simulink model "C172S_RollAttitudeHold_V1"  (R2026a)
settings: Solver=ode4  StartTime=0  StopTime=40  FixedStep=0.01
InitFcn:
  | rah1Data = c172sLateralDirectionalData();
  | [~,rah1Plant] = c172sLateralDirectionalPlant(rah1Data);
  | rah1YawController = c172sYawDamperData();
  | rah1RudderActuator = c172sRudderActuatorData();
  | rah1Controller = c172sRollAttitudeControllerData();
  | rah1AileronActuator = c172sAileronActuatorData();
  | if ~strcmp(rah1Data.model.version,rah1Controller.requiredPlantVersion), error('RAH V1 plant dependency mismatch.'); end
  | if ~strcmp(rah1YawController.artifactRevision,rah1Controller.requiredYawDamperRevision), error('RAH V1 yaw-controller dependency mismatch.'); end
  | if ~strcmp(rah1RudderActuator.artifactRevision,rah1Controller.requiredRudderAuditRevision), error('RAH V1 rudder-audit dependency mismatch.'); end
  | if ~strcmp(rah1AileronActuator.artifactRevision,rah1Controller.requiredAileronAuditRevision), error('RAH V1 aileron-audit dependency mismatch.'); end
  | A_rah1 = rah1Plant.A; B_rah1 = rah1Plant.B;
  | C_rah1 = rah1Plant.C; D_rah1 = rah1Plant.D;
  | Kphi_rah1 = rah1Controller.bankProportionalGain;
  | Ki_rah1 = rah1Controller.bankIntegralGain_per_s;
  | Kp_rah1 = rah1Controller.rollRateGain_s;
  | Tcmd_rah1 = rah1Controller.commandFilterTimeConstant_s;
  | Kr_rah1 = rah1YawController.rudderGain_s;
  | Tw_rah1 = rah1YawController.washoutTimeConstant_s;
  | TsRudder_rah1 = rah1RudderActuator.sensor.filterTimeConstant_s;
  | tauRudder_rah1 = rah1RudderActuator.dynamics.timeConstant_s;
  | TsRoll_rah1 = rah1AileronActuator.sensor.filterTimeConstant_s;
  | tauAileron_rah1 = rah1AileronActuator.dynamics.timeConstant_s;
  | Tt_rah1 = rah1AileronActuator.antiWindup.trackingTimeConstant_s;
  | delaySampleTime_rah1 = rah1AileronActuator.sensor.nominalDelay_s;
  | bankCommandLower_rah1_rad = rah1Controller.commandAuthority.lowerLimit_rad;
  | bankCommandUpper_rah1_rad = rah1Controller.commandAuthority.upperLimit_rad;
  | autoAileronLower_rah1_rad = rah1AileronActuator.authority.lowerLimit_rad;
  | autoAileronUpper_rah1_rad = rah1AileronActuator.authority.upperLimit_rad;
  | aileronRateLower_rah1_radps = -deg2rad(rah1AileronActuator.dynamics.rateLimit_degps);
  | aileronRateUpper_rah1_radps = deg2rad(rah1AileronActuator.dynamics.rateLimit_degps);
  | totalAileronLower_rah1_rad = rah1AileronActuator.physicalTravel.lowerLimit_rad;
  | totalAileronUpper_rah1_rad = rah1AileronActuator.physicalTravel.upperLimit_rad;
  | autoRudderLower_rah1_rad = rah1RudderActuator.authority.lowerLimit_rad;
  | autoRudderUpper_rah1_rad = rah1RudderActuator.authority.upperLimit_rad;
  | rudderRateLower_rah1_radps = -deg2rad(rah1RudderActuator.dynamics.rateLimit_degps);
  | rudderRateUpper_rah1_radps = deg2rad(rah1RudderActuator.dynamics.rateLimit_degps);
  | totalRudderLower_rah1_rad = rah1RudderActuator.physicalTravel.lowerLimit_rad;
  | totalRudderUpper_rah1_rad = rah1RudderActuator.physicalTravel.upperLimit_rad;
  | if ~exist('bankCommand_rah1_rad','var'), bankCommand_rah1_rad = deg2rad(10); end
  | if ~exist('pilotAileronBias_rah1_rad','var'), pilotAileronBias_rah1_rad = 0; end
  | if ~exist('pilotAileronPulse_rah1_rad','var'), pilotAileronPulse_rah1_rad = 0; end
  | if ~exist('pilotRudderBias_rah1_rad','var'), pilotRudderBias_rah1_rad = 0; end
  | if ~exist('pilotRudderPulse_rah1_rad','var'), pilotRudderPulse_rah1_rad = 0; end
  | if ~exist('aileronPulseStart_rah1_s','var'), aileronPulseStart_rah1_s = 5; end
  | if ~exist('aileronPulseEnd_rah1_s','var'), aileronPulseEnd_rah1_s = 6; end
  | if ~exist('rudderPulseStart_rah1_s','var'), rudderPulseStart_rah1_s = 5; end
  | if ~exist('rudderPulseEnd_rah1_s','var'), rudderPulseEnd_rah1_s = 6; end
  | if ~exist('pNoiseAmplitude_rah1_radps','var'), pNoiseAmplitude_rah1_radps = 0; end
  | if ~exist('pNoiseFrequency_rah1_radps','var'), pNoiseFrequency_rah1_radps = 50; end
  | if ~exist('phiNoiseAmplitude_rah1_rad','var'), phiNoiseAmplitude_rah1_rad = 0; end
  | if ~exist('phiNoiseFrequency_rah1_radps','var'), phiNoiseFrequency_rah1_radps = 5; end
  | if ~exist('yawNoiseAmplitude_rah1_radps','var'), yawNoiseAmplitude_rah1_radps = 0; end
  | if ~exist('yawNoiseFrequency_rah1_radps','var'), yawNoiseFrequency_rah1_radps = 50; end
  | if ~exist('antiWindupEnable_rah1','var'), antiWindupEnable_rah1 = 1; end
  | if ~exist('x0_rah1','var'), x0_rah1 = zeros(5,1); end
  | if ~exist('rDelay0_rah1_radps','var'), rDelay0_rah1_radps = x0_rah1(3); end
  | if ~exist('pDelay0_rah1_radps','var'), pDelay0_rah1_radps = x0_rah1(2); end
  | if ~exist('phiDelay0_rah1_rad','var'), phiDelay0_rah1_rad = x0_rah1(4); end
  | if ~exist('rSensor0_rah1_radps','var'), rSensor0_rah1_radps = 0; end
  | if ~exist('xw0_rah1_radps','var'), xw0_rah1_radps = 0; end
  | if ~exist('deltaRAuto0_rah1_rad','var'), deltaRAuto0_rah1_rad = 0; end
  | if ~exist('pSensor0_rah1_radps','var'), pSensor0_rah1_radps = 0; end
  | if ~exist('phiSensor0_rah1_rad','var'), phiSensor0_rah1_rad = 0; end
  | if ~exist('xi0_rah1_rad_s','var'), xi0_rah1_rad_s = 0; end
  | if ~exist('deltaAAuto0_rah1_rad','var'), deltaAAuto0_rah1_rad = 0; end
  | if ~exist('filteredCommand0_rah1_rad','var'), filteredCommand0_rah1_rad = 0; end
undefined symbols (not defined in the file or in its folder): aileronPulseEnd_rah1_s, aileronPulseStart_rah1_s, antiWindupEnable_rah1, deltaAAuto0_rah1_rad, deltaRAuto0_rah1_rad, filteredCommand0_rah1_rad, pDelay0_rah1_radps, phiDelay0_rah1_rad, phiNoiseAmplitude_rah1_rad, phiNoiseFrequency_rah1_radps, phiSensor0_rah1_rad, pilotAileronBias_rah1_rad, pilotAileronPulse_rah1_rad, pilotRudderBias_rah1_rad, pilotRudderPulse_rah1_rad, pNoiseAmplitude_rah1_radps, pNoiseFrequency_rah1_radps, pSensor0_rah1_radps, rDelay0_rah1_radps, rSensor0_rah1_radps, rudderPulseEnd_rah1_s, rudderPulseStart_rah1_s, x0_rah1, xi0_rah1_rad_s, xw0_rah1_radps, yawNoiseAmplitude_rah1_radps, yawNoiseFrequency_rah1_radps
settings Model: Creator=Shahi  LastModifiedBy=Shahi

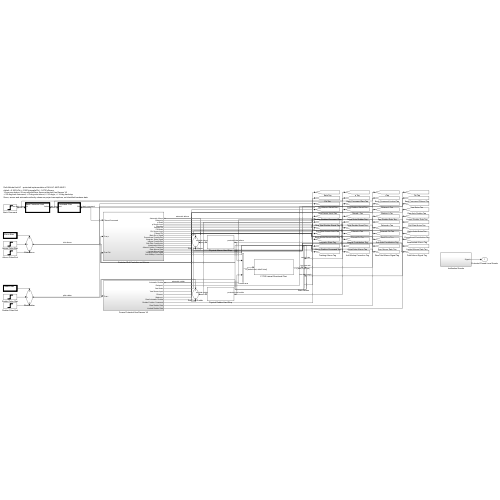
[thumbnail: Simulink's stored preview of the top-level diagram]
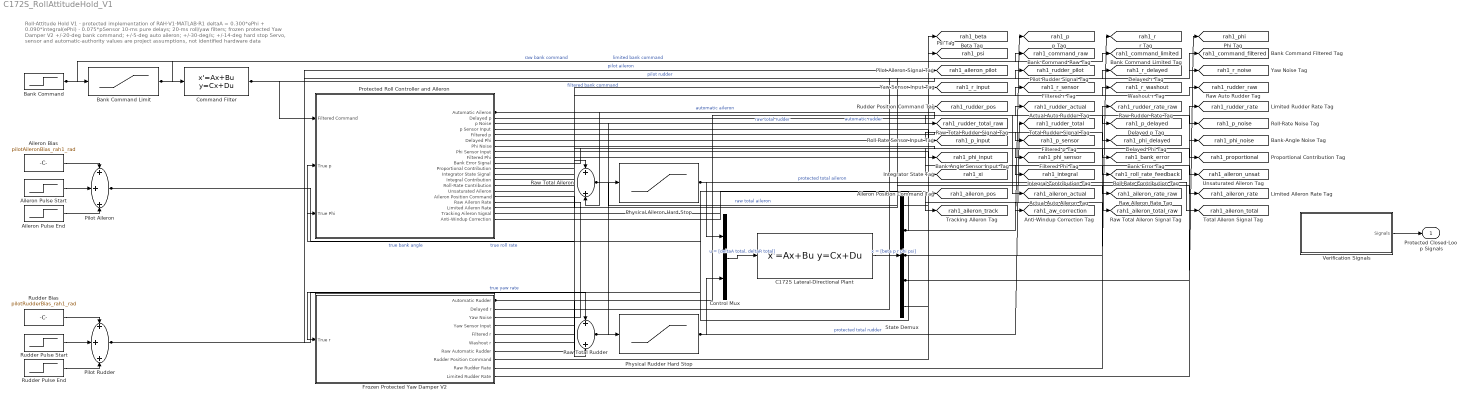
== system C172S_RollAttitudeHold_V1 ==
  note: Roll-Attitude Hold V1 - protected implementation of RAH-V1-MATLAB-R1
      | deltaA = 0.300*ePhi + 0.090*integral(ePhi) - 0.075*pSensor
      | 10-ms pure delays; 20-ms roll/yaw filters; frozen protected Yaw Damper V2
      | +/-20-deg bank command; +/-5-deg auto aileron; +/-30-deg/s; +/-14-deg hard stop
      | Servo, sensor and automatic-authority values are project assumptions, not identified hardware data
  Aileron Bias : Constant  Value=pilotAileronBias_rah1_rad
  Aileron Pulse End : Step  Time=aileronPulseEnd_rah1_s  FinalValue=-pilotAileronPulse_rah1_rad  SampleTime=0
  Aileron Pulse Start : Step  Time=aileronPulseStart_rah1_s  FinalValue=pilotAileronPulse_rah1_rad  SampleTime=0
  Bank Command : Step  Time=0  FinalValue=bankCommand_rah1_rad  SampleTime=0
  Bank Command Limit : Saturate  UpperLimit=bankCommandUpper_rah1_rad  LowerLimit=bankCommandLower_rah1_rad
  C172S Lateral-Directional Plant : StateSpace  A=A_rah1  B=B_rah1  C=C_rah1  D=D_rah1  InitialCondition=x0_rah1
  Command Filter : StateSpace  A=-1/Tcmd_rah1  B=1/Tcmd_rah1  D=0  InitialCondition=filteredCommand0_rah1_rad
  Control Mux : Mux  Inputs=2
  Frozen Protected Yaw Damper V2 : Subsystem
  Physical Aileron Hard Stop : Saturate  UpperLimit=totalAileronUpper_rah1_rad  LowerLimit=totalAileronLower_rah1_rad
  Physical Rudder Hard Stop : Saturate  UpperLimit=totalRudderUpper_rah1_rad  LowerLimit=totalRudderLower_rah1_rad
  Pilot Aileron : Sum  Inputs=+++
  Pilot Rudder : Sum  Inputs=+++
  Protected Roll Controller and Aileron : Subsystem
  Raw Total Aileron : Sum
  Raw Total Rudder : Sum
  Rudder Bias : Constant  Value=pilotRudderBias_rah1_rad
  Rudder Pulse End : Step  Time=rudderPulseEnd_rah1_s  FinalValue=-pilotRudderPulse_rah1_rad  SampleTime=0
  Rudder Pulse Start : Step  Time=rudderPulseStart_rah1_s  FinalValue=pilotRudderPulse_rah1_rad  SampleTime=0
  State Demux : Demux  Outputs=5
  Verification Signals : Subsystem
  Protected Closed-Loop Signals : Outport
  tag scope: rah1_aileron_actual=global, rah1_aileron_pilot=global, rah1_aileron_pos=global, rah1_aileron_rate=global, rah1_aileron_rate_raw=global, rah1_aileron_total=global, rah1_aileron_total_raw=global, rah1_aileron_track=global, rah1_aileron_unsat=global, rah1_aw_correction=global, rah1_bank_error=global, rah1_beta=global, rah1_command_filtered=global, rah1_command_limited=global, rah1_command_raw=global, rah1_integral=global, rah1_p=global, rah1_p_delayed=global, rah1_p_input=global, rah1_p_noise=global, rah1_p_sensor=global, rah1_phi=global, rah1_phi_delayed=global, rah1_phi_input=global, rah1_phi_noise=global, rah1_phi_sensor=global, rah1_proportional=global, rah1_psi=global, rah1_r=global, rah1_r_delayed=global, rah1_r_input=global, rah1_r_noise=global, rah1_r_sensor=global, rah1_r_washout=global, rah1_roll_rate_feedback=global, rah1_rudder_actual=global, rah1_rudder_pilot=global, rah1_rudder_pos=global, rah1_rudder_rate=global, rah1_rudder_rate_raw=global, rah1_rudder_raw=global, rah1_rudder_total=global, rah1_rudder_total_raw=global, rah1_xi=global
  wires:
  Bank Command/1 -> Bank Command Limit/1, [rah1_command_raw]  "raw bank command"
  Bank Command Limit/1 -> Command Filter/1, [rah1_command_limited]  "limited bank command"
  Command Filter/1 -> Protected Roll Controller and Aileron/1(Filtered Command), [rah1_command_filtered]  "filtered bank command"
  Aileron Bias/1 -> Pilot Aileron/1
  Aileron Pulse Start/1 -> Pilot Aileron/2
  Aileron Pulse End/1 -> Pilot Aileron/3
  Rudder Bias/1 -> Pilot Rudder/1
  Rudder Pulse Start/1 -> Pilot Rudder/2
  Rudder Pulse End/1 -> Pilot Rudder/3
  Pilot Aileron/1 -> Raw Total Aileron/1, [rah1_aileron_pilot]  "pilot aileron"
  Protected Roll Controller and Aileron/1(Automatic Aileron) -> Raw Total Aileron/2, [rah1_aileron_actual]  "automatic aileron"
  Raw Total Aileron/1 -> Physical Aileron Hard Stop/1, [rah1_aileron_total_raw]  "raw total aileron"
  Physical Aileron Hard Stop/1 -> Control Mux/1, [rah1_aileron_total]  "protected total aileron"
  Pilot Rudder/1 -> Raw Total Rudder/1, [rah1_rudder_pilot]  "pilot rudder"
  Frozen Protected Yaw Damper V2/1(Automatic Rudder) -> Raw Total Rudder/2, [rah1_rudder_actual]  "automatic rudder"
  Raw Total Rudder/1 -> Physical Rudder Hard Stop/1, [rah1_rudder_total_raw]  "raw total rudder"
  Physical Rudder Hard Stop/1 -> Control Mux/2, [rah1_rudder_total]  "protected total rudder"
  Control Mux/1 -> C172S Lateral-Directional Plant/1  "u = [deltaA total, deltaR total]"
  C172S Lateral-Directional Plant/1 -> State Demux/1  "x = [beta p r phi psi]"
  State Demux/2 -> Protected Roll Controller and Aileron/2(True p), [rah1_p]  "true roll rate"
  State Demux/4 -> Protected Roll Controller and Aileron/3(True Phi), [rah1_phi]  "true bank angle"
  State Demux/3 -> Frozen Protected Yaw Damper V2/1(True r), [rah1_r]  "true yaw rate"
  Verification Signals/1(Signals) -> Protected Closed-Loop Signals/1
  State Demux/1 -> [rah1_beta]
  State Demux/5 -> [rah1_psi]
  Frozen Protected Yaw Damper V2/2(Delayed r) -> [rah1_r_delayed]
  Frozen Protected Yaw Damper V2/3(Yaw Noise) -> [rah1_r_noise]
  Frozen Protected Yaw Damper V2/4(Yaw Sensor Input) -> [rah1_r_input]
  Frozen Protected Yaw Damper V2/5(Filtered r) -> [rah1_r_sensor]
  Frozen Protected Yaw Damper V2/6(Washout r) -> [rah1_r_washout]
  Frozen Protected Yaw Damper V2/7(Raw Automatic Rudder) -> [rah1_rudder_raw]
  Frozen Protected Yaw Damper V2/8(Rudder Position Command) -> [rah1_rudder_pos]
  Frozen Protected Yaw Damper V2/9(Raw Rudder Rate) -> [rah1_rudder_rate_raw]
  Frozen Protected Yaw Damper V2/10(Limited Rudder Rate) -> [rah1_rudder_rate]
  Protected Roll Controller and Aileron/2(Delayed p) -> [rah1_p_delayed]
  Protected Roll Controller and Aileron/3(p Noise) -> [rah1_p_noise]
  Protected Roll Controller and Aileron/4(p Sensor Input) -> [rah1_p_input]
  Protected Roll Controller and Aileron/5(Filtered p) -> [rah1_p_sensor]
  Protected Roll Controller and Aileron/6(Delayed Phi) -> [rah1_phi_delayed]
  Protected Roll Controller and Aileron/7(Phi Noise) -> [rah1_phi_noise]
  Protected Roll Controller and Aileron/8(Phi Sensor Input) -> [rah1_phi_input]
  Protected Roll Controller and Aileron/9(Filtered Phi) -> [rah1_phi_sensor]
  Protected Roll Controller and Aileron/10(Bank Error Signal) -> [rah1_bank_error]
  Protected Roll Controller and Aileron/11(Proportional Contribution) -> [rah1_proportional]
  Protected Roll Controller and Aileron/12(Integrator State Signal) -> [rah1_xi]
  Protected Roll Controller and Aileron/13(Integral Contribution) -> [rah1_integral]
  Protected Roll Controller and Aileron/14(Roll-Rate Contribution) -> [rah1_roll_rate_feedback]
  Protected Roll Controller and Aileron/15(Unsaturated Aileron) -> [rah1_aileron_unsat]
  Protected Roll Controller and Aileron/16(Aileron Position Command) -> [rah1_aileron_pos]
  Protected Roll Controller and Aileron/17(Raw Aileron Rate) -> [rah1_aileron_rate_raw]
  Protected Roll Controller and Aileron/18(Limited Aileron Rate) -> [rah1_aileron_rate]
  Protected Roll Controller and Aileron/19(Tracking Aileron Signal) -> [rah1_aileron_track]
  Protected Roll Controller and Aileron/20(Anti-Windup Correction) -> [rah1_aw_correction]

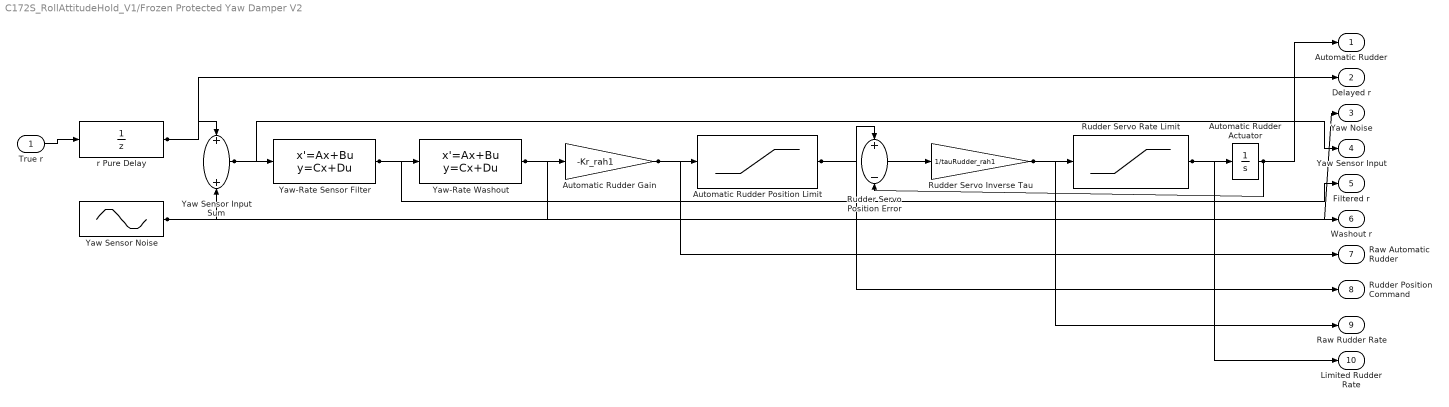
== system C172S_RollAttitudeHold_V1/Frozen Protected Yaw Damper V2 ==
  True r : Inport
  Automatic Rudder Actuator : Integrator  InitialCondition=deltaRAuto0_rah1_rad
  Automatic Rudder Gain : Gain  Gain=-Kr_rah1
  Automatic Rudder Position Limit : Saturate  UpperLimit=autoRudderUpper_rah1_rad  LowerLimit=autoRudderLower_rah1_rad
  Rudder Servo Inverse Tau : Gain  Gain=1/tauRudder_rah1
  Rudder Servo Position Error : Sum  Inputs=+-
  Rudder Servo Rate Limit : Saturate  UpperLimit=rudderRateUpper_rah1_radps  LowerLimit=rudderRateLower_rah1_radps
  Yaw Sensor Input Sum : Sum
  Yaw Sensor Noise : Sin  Amplitude=yawNoiseAmplitude_rah1_radps  Frequency=yawNoiseFrequency_rah1_radps  SampleTime=0
  Yaw-Rate Sensor Filter : StateSpace  A=-1/TsRudder_rah1  B=1/TsRudder_rah1  D=0  InitialCondition=rSensor0_rah1_radps
  Yaw-Rate Washout : StateSpace  A=-1/Tw_rah1  B=1/Tw_rah1  C=-1  InitialCondition=xw0_rah1_radps
  r Pure Delay : UnitDelay  InitialCondition=rDelay0_rah1_radps  SampleTime=delaySampleTime_rah1
  Automatic Rudder : Outport
  Delayed r : Outport  Port=2
  Yaw Noise : Outport  Port=3
  Yaw Sensor Input : Outport  Port=4
  Filtered r : Outport  Port=5
  Washout r : Outport  Port=6
  Raw Automatic Rudder : Outport  Port=7
  Rudder Position Command : Outport  Port=8
  Raw Rudder Rate : Outport  Port=9
  Limited Rudder Rate : Outport  Port=10
  wires:
  True r/1 -> r Pure Delay/1
  r Pure Delay/1 -> Yaw Sensor Input Sum/1, Delayed r/1
  Yaw Sensor Noise/1 -> Yaw Sensor Input Sum/2, Yaw Noise/1
  Yaw Sensor Input Sum/1 -> Yaw-Rate Sensor Filter/1, Yaw Sensor Input/1
  Yaw-Rate Sensor Filter/1 -> Yaw-Rate Washout/1, Filtered r/1
  Yaw-Rate Washout/1 -> Automatic Rudder Gain/1, Washout r/1
  Automatic Rudder Gain/1 -> Automatic Rudder Position Limit/1, Raw Automatic Rudder/1
  Automatic Rudder Position Limit/1 -> Rudder Servo Position Error/1, Rudder Position Command/1
  Automatic Rudder Actuator/1 -> Rudder Servo Position Error/2, Automatic Rudder/1
  Rudder Servo Position Error/1 -> Rudder Servo Inverse Tau/1
  Rudder Servo Inverse Tau/1 -> Rudder Servo Rate Limit/1, Raw Rudder Rate/1
  Rudder Servo Rate Limit/1 -> Automatic Rudder Actuator/1, Limited Rudder Rate/1

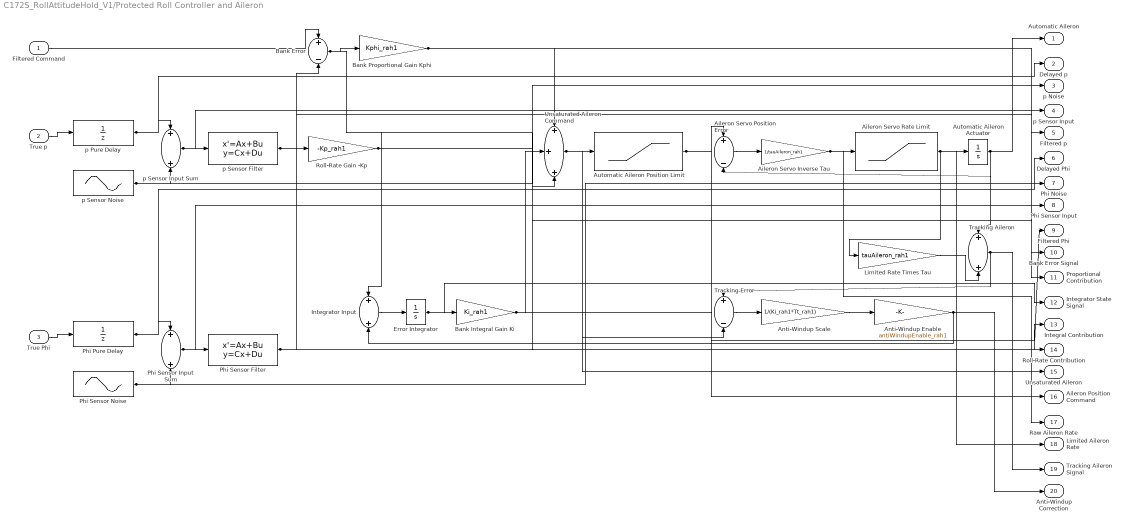
== system C172S_RollAttitudeHold_V1/Protected Roll Controller and Aileron ==
  Filtered Command : Inport
  True p : Inport  Port=2
  True Phi : Inport  Port=3
  Aileron Servo Inverse Tau : Gain  Gain=1/tauAileron_rah1
  Aileron Servo Position Error : Sum  Inputs=+-
  Aileron Servo Rate Limit : Saturate  UpperLimit=aileronRateUpper_rah1_radps  LowerLimit=aileronRateLower_rah1_radps
  Anti-Windup Enable : Gain  Gain=antiWindupEnable_rah1
  Anti-Windup Scale : Gain  Gain=1/(Ki_rah1*Tt_rah1)
  Automatic Aileron Actuator : Integrator  InitialCondition=deltaAAuto0_rah1_rad
  Automatic Aileron Position Limit : Saturate  UpperLimit=autoAileronUpper_rah1_rad  LowerLimit=autoAileronLower_rah1_rad
  Bank Error : Sum  Inputs=+-
  Bank Integral Gain Ki : Gain  Gain=Ki_rah1
  Bank Proportional Gain Kphi : Gain  Gain=Kphi_rah1
  Error Integrator : Integrator  InitialCondition=xi0_rah1_rad_s
  Integrator Input : Sum
  Limited Rate Times Tau : Gain  Gain=tauAileron_rah1
  Phi Pure Delay : UnitDelay  InitialCondition=phiDelay0_rah1_rad  SampleTime=delaySampleTime_rah1
  Phi Sensor Filter : StateSpace  A=-1/TsRoll_rah1  B=1/TsRoll_rah1  D=0  InitialCondition=phiSensor0_rah1_rad
  Phi Sensor Input Sum : Sum
  Phi Sensor Noise : Sin  Amplitude=phiNoiseAmplitude_rah1_rad  Frequency=phiNoiseFrequency_rah1_radps  SampleTime=0
  Roll-Rate Gain -Kp : Gain  Gain=-Kp_rah1
  Tracking Aileron : Sum
  Tracking Error : Sum  Inputs=+-
  Unsaturated Aileron Command : Sum  Inputs=+++
  p Pure Delay : UnitDelay  InitialCondition=pDelay0_rah1_radps  SampleTime=delaySampleTime_rah1
  p Sensor Filter : StateSpace  A=-1/TsRoll_rah1  B=1/TsRoll_rah1  D=0  InitialCondition=pSensor0_rah1_radps
  p Sensor Input Sum : Sum
  p Sensor Noise : Sin  Amplitude=pNoiseAmplitude_rah1_radps  Frequency=pNoiseFrequency_rah1_radps  SampleTime=0
  Automatic Aileron : Outport
  Delayed p : Outport  Port=2
  p Noise : Outport  Port=3
  p Sensor Input : Outport  Port=4
  Filtered p : Outport  Port=5
  Delayed Phi : Outport  Port=6
  Phi Noise : Outport  Port=7
  Phi Sensor Input : Outport  Port=8
  Filtered Phi : Outport  Port=9
  Bank Error Signal : Outport  Port=10
  Proportional Contribution : Outport  Port=11
  Integrator State Signal : Outport  Port=12
  Integral Contribution : Outport  Port=13
  Roll-Rate Contribution : Outport  Port=14
  Unsaturated Aileron : Outport  Port=15
  Aileron Position Command : Outport  Port=16
  Raw Aileron Rate : Outport  Port=17
  Limited Aileron Rate : Outport  Port=18
  Tracking Aileron Signal : Outport  Port=19
  Anti-Windup Correction : Outport  Port=20
  wires:
  True p/1 -> p Pure Delay/1
  p Pure Delay/1 -> p Sensor Input Sum/1, Delayed p/1
  p Sensor Noise/1 -> p Sensor Input Sum/2, p Noise/1
  p Sensor Input Sum/1 -> p Sensor Filter/1, p Sensor Input/1
  p Sensor Filter/1 -> Roll-Rate Gain -Kp/1, Filtered p/1
  True Phi/1 -> Phi Pure Delay/1
  Phi Pure Delay/1 -> Phi Sensor Input Sum/1, Delayed Phi/1
  Phi Sensor Noise/1 -> Phi Sensor Input Sum/2, Phi Noise/1
  Phi Sensor Input Sum/1 -> Phi Sensor Filter/1, Phi Sensor Input/1
  Filtered Command/1 -> Bank Error/1
  Phi Sensor Filter/1 -> Bank Error/2, Filtered Phi/1
  Bank Error/1 -> Bank Proportional Gain Kphi/1, Integrator Input/1, Bank Error Signal/1
  Integrator Input/1 -> Error Integrator/1
  Error Integrator/1 -> Bank Integral Gain Ki/1, Integrator State Signal/1
  Bank Proportional Gain Kphi/1 -> Unsaturated Aileron Command/1, Proportional Contribution/1
  Bank Integral Gain Ki/1 -> Unsaturated Aileron Command/2, Integral Contribution/1
  Roll-Rate Gain -Kp/1 -> Unsaturated Aileron Command/3, Roll-Rate Contribution/1
  Unsaturated Aileron Command/1 -> Automatic Aileron Position Limit/1, Tracking Error/2, Unsaturated Aileron/1
  Automatic Aileron Position Limit/1 -> Aileron Servo Position Error/1, Aileron Position Command/1
  Automatic Aileron Actuator/1 -> Aileron Servo Position Error/2, Tracking Aileron/1, Automatic Aileron/1
  Aileron Servo Position Error/1 -> Aileron Servo Inverse Tau/1
  Aileron Servo Inverse Tau/1 -> Aileron Servo Rate Limit/1, Raw Aileron Rate/1
  Aileron Servo Rate Limit/1 -> Automatic Aileron Actuator/1, Limited Rate Times Tau/1, Limited Aileron Rate/1
  Limited Rate Times Tau/1 -> Tracking Aileron/2
  Tracking Aileron/1 -> Tracking Error/1, Tracking Aileron Signal/1
  Tracking Error/1 -> Anti-Windup Scale/1
  Anti-Windup Scale/1 -> Anti-Windup Enable/1
  Anti-Windup Enable/1 -> Integrator Input/2, Anti-Windup Correction/1

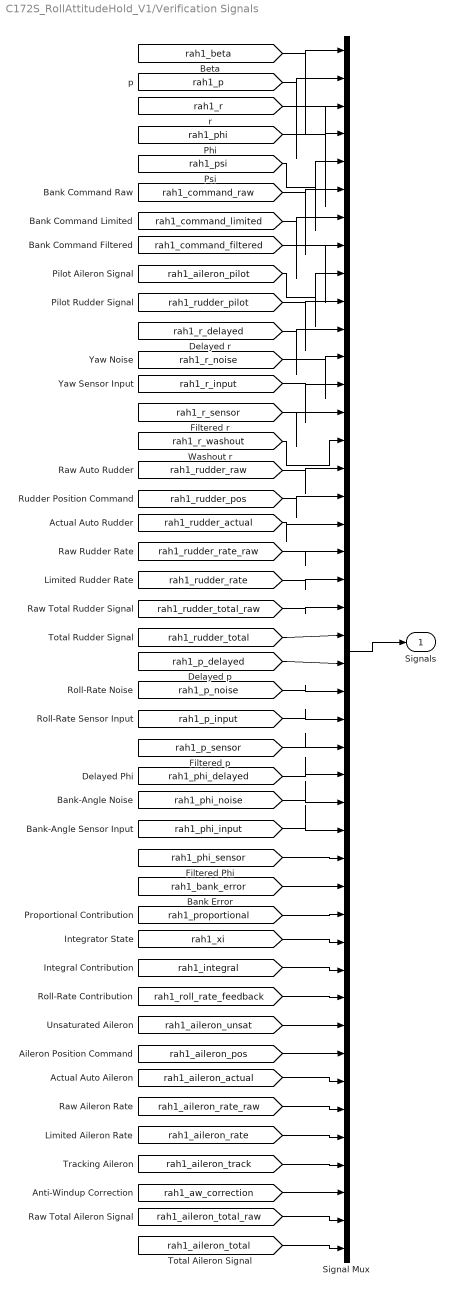
== system C172S_RollAttitudeHold_V1/Verification Signals ==
  Signal Mux : Mux  Inputs=44
  Signals : Outport
  wires:
  [rah1_beta] -> Signal Mux/1
  [rah1_p] -> Signal Mux/2
  [rah1_r] -> Signal Mux/3
  [rah1_phi] -> Signal Mux/4
  [rah1_psi] -> Signal Mux/5
  [rah1_command_raw] -> Signal Mux/6
  [rah1_command_limited] -> Signal Mux/7
  [rah1_command_filtered] -> Signal Mux/8
  [rah1_aileron_pilot] -> Signal Mux/9
  [rah1_rudder_pilot] -> Signal Mux/10
  [rah1_r_delayed] -> Signal Mux/11
  [rah1_r_noise] -> Signal Mux/12
  [rah1_r_input] -> Signal Mux/13
  [rah1_r_sensor] -> Signal Mux/14
  [rah1_r_washout] -> Signal Mux/15
  [rah1_rudder_raw] -> Signal Mux/16
  [rah1_rudder_pos] -> Signal Mux/17
  [rah1_rudder_actual] -> Signal Mux/18
  [rah1_rudder_rate_raw] -> Signal Mux/19
  [rah1_rudder_rate] -> Signal Mux/20
  [rah1_rudder_total_raw] -> Signal Mux/21
  [rah1_rudder_total] -> Signal Mux/22
  [rah1_p_delayed] -> Signal Mux/23
  [rah1_p_noise] -> Signal Mux/24
  [rah1_p_input] -> Signal Mux/25
  [rah1_p_sensor] -> Signal Mux/26
  [rah1_phi_delayed] -> Signal Mux/27
  [rah1_phi_noise] -> Signal Mux/28
  [rah1_phi_input] -> Signal Mux/29
  [rah1_phi_sensor] -> Signal Mux/30
  [rah1_bank_error] -> Signal Mux/31
  [rah1_proportional] -> Signal Mux/32
  [rah1_xi] -> Signal Mux/33
  [rah1_integral] -> Signal Mux/34
  [rah1_roll_rate_feedback] -> Signal Mux/35
  [rah1_aileron_unsat] -> Signal Mux/36
  [rah1_aileron_pos] -> Signal Mux/37
  [rah1_aileron_actual] -> Signal Mux/38
  [rah1_aileron_rate_raw] -> Signal Mux/39
  [rah1_aileron_rate] -> Signal Mux/40
  [rah1_aileron_track] -> Signal Mux/41
  [rah1_aw_correction] -> Signal Mux/42
  [rah1_aileron_total_raw] -> Signal Mux/43
  [rah1_aileron_total] -> Signal Mux/44
  Signal Mux/1 -> Signals/1
